simulink library "foc"  (Simulink 8.1)
settings: Solver=ode1  StartTime=0.0  StopTime=Inf  FixedStep=0.001  RelTol=1e-3
PostLoadFcn:
  | , if any(exist('dsrtsu_mdlpostloadfcn', 'file') == [2, 3, 6]), try dsrtsu_mdlpostloadfcn('Execute', bdroot); catch fprintf('Error in PostLoadFcn (dsrtsu_mdlpostloadfcn) for model "%s":\n %s\n', bdroot, lasterr); end, end,
settings Model: DSRTSU_INTERNAL_RTI_VER=450  DSRTSU_INTERNAL_RTI_TYPE=rti1401  RTICANMMDATA=struct('GeneralSetupData',struct('modelroot','D:\Soichi\SVNDATA\IDIADA_ADAS\trunk\AdasDragon\software\sw_development\arch\app\jud','generalsettings',struct('filesettings',struct('destfolder',struct('Name','RTICANMM_FILES','Check',1),'buildfolder',struct('Name','.','Check',1),'AbsDestfolder',struct('Name','D:\Soichi\SVNDATA\IDIADA_ADAS\trunk\AdasDragon\software\sw_development\arch\app\jud\RTICANMM_FILES'),'AbsBuildfolder',struct('Name','D:\Soichi\SVNDATA\IDIADA_ADAS\trunk\AdasDragon\software\sw_development\arch\app\jud'))),'options',struct('addpaths',1,'rmpaths',1,'addtrcexclusion',logical(1),'cannavigator',struct('checkmonitoring',0),'show_usrtrc',0,'use_usrtrc',0),'advanced',struct('options',[1 1 1 1 1 1 1 1 1 1 1 1 1 1 1 1 1 1 1 1 1 1 1 1 1 1 1 1 1 1 1 1 1 1 1 1 1 1 1 1 1 1 1 1 1 1 1 1 1 1 1 1 1 1 1 1 1 1 1 1 1 1 1 1 1 1 1 1 1 1 1 1 1 1 1 1 1 1 1 1 1 1 1 1 1 1 1 1 1 1 1 1 1 1 1 1 1 1 1 1]),'MPSetup',{{}},'modelname','foc','block','foc'))  DSRTSU_INTERNAL_RTIFPGA=40  Creator=AT015411  LastModifiedBy=AT015411

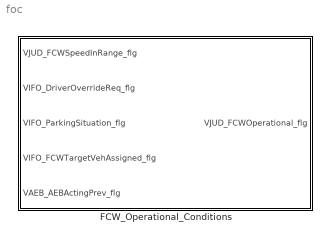
== system foc ==
  FCW_Operational_Conditions : Subsystem

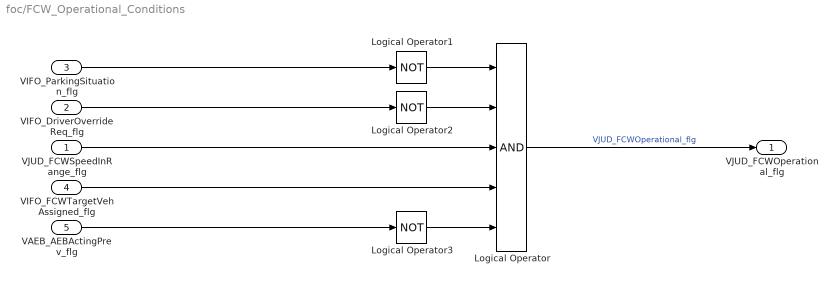
== system foc/FCW_Operational_Conditions ==
  VJUD_FCWSpeedInRange_flg : Inport
  VIFO_DriverOverrideReq_flg : Inport  Port=2
  VIFO_ParkingSituation_flg : Inport  Port=3
  VIFO_FCWTargetVehAssigned_flg : Inport  Port=4
  VAEB_AEBActingPrev_flg : Inport  Port=5
  Logical Operator : Logic  Inputs=5  AllPortsSameDT=off  OutDataTypeStr=boolean
  Logical Operator1 : Logic  Operator=NOT  AllPortsSameDT=off  OutDataTypeStr=boolean
  Logical Operator2 : Logic  Operator=NOT  AllPortsSameDT=off  OutDataTypeStr=boolean
  Logical Operator3 : Logic  Operator=NOT  AllPortsSameDT=off  OutDataTypeStr=boolean
  VJUD_FCWOperational_flg : Outport
  wires:
  VJUD_FCWSpeedInRange_flg/1 -> Logical Operator/3
  VIFO_ParkingSituation_flg/1 -> Logical Operator1/1
  VIFO_DriverOverrideReq_flg/1 -> Logical Operator2/1
  Logical Operator1/1 -> Logical Operator/1
  Logical Operator2/1 -> Logical Operator/2
  Logical Operator/1 -> VJUD_FCWOperational_flg/1  "VJUD_FCWOperational_flg"
  VIFO_FCWTargetVehAssigned_flg/1 -> Logical Operator/4
  VAEB_AEBActingPrev_flg/1 -> Logical Operator3/1
  Logical Operator3/1 -> Logical Operator/5
